simulink model "CarOnBump"  (Simulink 8.5)
settings: Solver=ode45  StartTime=0.0  StopTime=18  RelTol=1e-3
libraries: vrlib x1
settings Model: Creator=User  LastModifiedBy=User
settings DataIOCC: SignalLoggingSaveFormat=Dataset
settings OptimizationCC: ExpressionDepthLimit=128
settings DebuggingCC: UnderspecifiedInitializationDetection=Simplified  MergeDetectMultiDrivingBlocksExec=error  FcnCallInpInsideContextMsg=EnableAllAsError  StateNameClashWarn=none
settings GRTTargetCC: CombineOutputUpdateFcns=on  GRTInterface=off

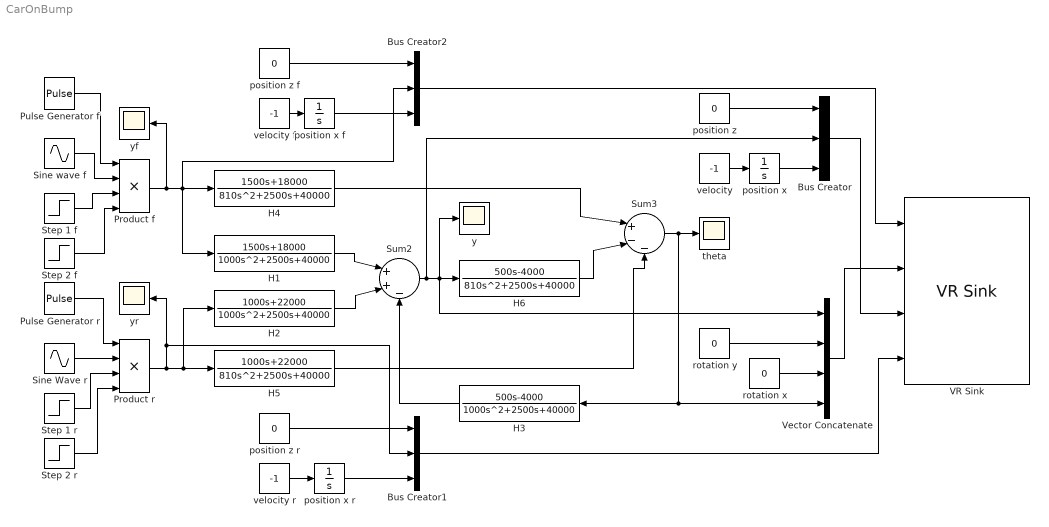
== system CarOnBump ==
  Bus Creator : BusCreator  Inputs=3
  Bus Creator1 : BusCreator  Inputs=3
  Bus Creator2 : BusCreator  Inputs=3
  H1 : TransferFcn  Numerator=[1500 18000]  Denominator=[1000 2500 40000]
  H2 : TransferFcn  Numerator=[1000 22000]  Denominator=[1000 2500 40000]
  H3 : TransferFcn  Numerator=[500 -4000]  Denominator=[1000 2500 40000]
  H4 : TransferFcn  Numerator=[1500 18000]  Denominator=[810 2500 40000]
  H5 : TransferFcn  Numerator=[1000 22000]  Denominator=[810 2500 40000]
  H6 : TransferFcn  Numerator=[500 -4000]  Denominator=[810 2500 40000]
  Product f : Product  Inputs=4
  "Product r " : Product  Inputs=4
  Pulse Generator f : DiscretePulseGenerator  PulseType=Time based  PulseWidth=50
  Pulse Generator r : DiscretePulseGenerator  PulseType=Time based  PulseWidth=50
  Sine Wave r : Sin  Amplitude=0.4  Frequency=pi  SampleTime=0
  Sine wave f : Sin  Amplitude=0.4  Frequency=pi  Phase=-2*pi  SampleTime=0
  Step 1 f : Step  Time=7.5  Before=1  After=0  SampleTime=0
  Step 1 r : Step  Time=9.5  Before=1  After=0  SampleTime=0
  Step 2 f : Step  Time=5.5  SampleTime=0
  Step 2 r : Step  Time=7.5  SampleTime=0
  Sum2 : Sum  Inputs=|++-
  Sum3 : Sum  Inputs=|+--
  VR Sink : vrlib/VR Sink  InstantiateOnLoad=on  SampleTime=0.05  ViewEnable=on  RemoteChange=off  RemoteView=off  FieldsWritten=front_wheels.translation.3.1.1.double#body.rotation.4.1.1.double#body.translation.3.1.1.double#rear_wheels.translation.3.1.1.double  WorldFileName=car.wrl  AutoView=off  VideoDimensions=[]  AllowVariableSize=off
  Vector Concatenate : Concatenate  NumInputs=4
  position x : Integrator
  position x f : Integrator
  position x r : Integrator
  position z : Constant  Value=0
  position z f : Constant  Value=0
  position z r : Constant  Value=0
  rotation x : Constant  Value=0
  rotation y : Constant  Value=0
  theta : Scope
      settings: TimeRange=16  YMin=-0.3  YMax=0.3  SaveName=ScopeData4
  velocity : Constant  Value=-1
  velocity f : Constant  Value=-1
  velocity r : Constant  Value=-1
  y : Scope
      settings: TimeRange=16  YMin=-0.2  YMax=0.3  SaveName=ScopeData3
  yf : Scope
      settings: TimeRange=18  YMin=-1.959434878635765e-16  YMax=0.4  SaveName=ScopeData5
  yr : Scope
      settings: TimeRange=18  YMin=-3.918869757271531e-16  YMax=0.4  SaveName=ScopeData6
  wires:
  Sine Wave r/1 -> "Product r "/2
  Pulse Generator r/1 -> "Product r "/1
  Sine wave f/1 -> Product f/2
  Pulse Generator f/1 -> Product f/1
  Product f/1 -> yf/1, Bus Creator2/2, H1/1, H4/1
  H1/1 -> Sum2/1
  H2/1 -> Sum2/2
  Sum2/1 -> Vector Concatenate/1, H6/1, y/1, Bus Creator/2
  H5/1 -> Sum3/3
  H6/1 -> Sum3/2
  H4/1 -> Sum3/1
  H3/1 -> Sum2/3
  position z/1 -> Bus Creator/1
  velocity/1 -> position x/1
  position x/1 -> Bus Creator/3
  rotation x/1 -> Vector Concatenate/3
  rotation y/1 -> Vector Concatenate/2
  Step 1 r/1 -> "Product r "/3
  Step 2 r/1 -> "Product r "/4
  Step 1 f/1 -> Product f/3
  Step 2 f/1 -> Product f/4
  "Product r "/1 -> Bus Creator1/2, yr/1, H5/1, H2/1
  position z r/1 -> Bus Creator1/1
  velocity r/1 -> position x r/1
  position x r/1 -> Bus Creator1/3
  position z f/1 -> Bus Creator2/1
  velocity f/1 -> position x f/1
  position x f/1 -> Bus Creator2/3
  Sum3/1 -> Vector Concatenate/4, H3/1, theta/1
  Vector Concatenate/1 -> VR Sink/2
  Bus Creator/1 -> VR Sink/3
  Bus Creator1/1 -> VR Sink/4
  Bus Creator2/1 -> VR Sink/1
